simulink model "gain_scheduling_sm_2_lookuptable_WP5_seno_frequenza_1"  (R2023b)
settings: Solver=VariableStepAuto  StartTime=0.0  StopTime=10  RelTol=1e-3
values from neighbouring files (symbols this model uses):
  k1_sigma = [k1_sigma,double(subs(gains.k1, 'sigma', i))]    [gain_sheduling_WP5.m]
  k2_sigma = [k2_sigma,double(subs(gains.k2, 'sigma', i))]    [gain_sheduling_WP5.m]
  sigma = input(1)    [GS_compute_gains_LQI.m]    (also in GS_compute_gains_LQR.m; GS_compute_gains_PP.m = rif; compute_gains_WP5.m = rif; gain_sheduling_WP5.m = [-pi+pi/16:pi/16:pi])
settings Model: Creator=miche  LastModifiedBy=miche

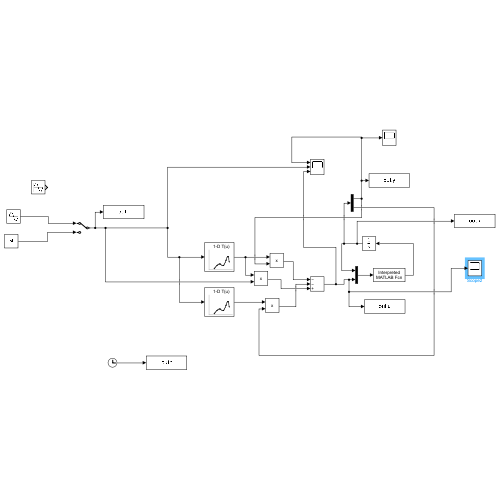
[thumbnail: Simulink's stored preview of the top-level diagram]
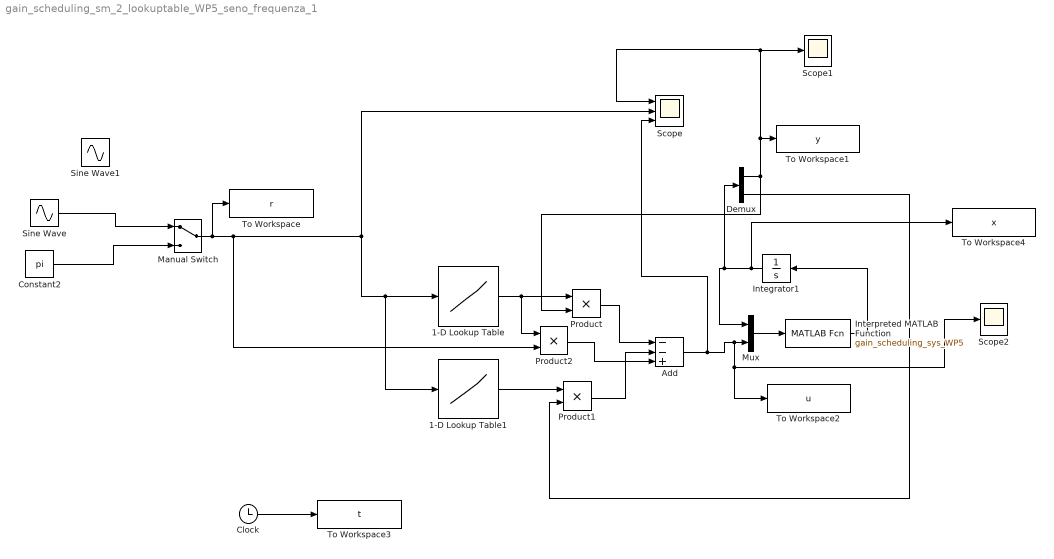
== system gain_scheduling_sm_2_lookuptable_WP5_seno_frequenza_1 ==
  1-D Lookup Table : Lookup_n-D  NumberOfTableDimensions=1  BreakpointsForDimension1=sigma  Table=k1_sigma  InterpMethod=Cubic spline  InternalRulePriority=Speed  RndMeth=Simplest
  1-D Lookup Table1 : Lookup_n-D  NumberOfTableDimensions=1  BreakpointsForDimension1=sigma  Table=k2_sigma  InterpMethod=Cubic spline  InternalRulePriority=Speed  RndMeth=Simplest
  Add : Sum  Inputs=--+
  Clock : Clock
  Constant2 : Constant  Value=pi
  Demux : Demux  Outputs=2
  Integrator1 : Integrator
  Interpreted MATLAB Function : MATLABFcn  MATLABFcn=gain_scheduling_sys_WP5  OutputDimensions=2
  Manual Switch : ManualSwitch
  Mux : Mux  Inputs=2
  Product : Product
  Product1 : Product
  Product2 : Product
  Scope : Scope  NumInputPorts=3
  Scope1 : Scope
  Scope2 : Scope
  Sine Wave : Sin  Amplitude=3.14  SampleTime=0
  Sine Wave1 : Sin  SampleTime=0
  To Workspace : ToWorkspace  VariableName=r  SampleTime=-1
  To Workspace1 : ToWorkspace  VariableName=y  SampleTime=-1
  To Workspace2 : ToWorkspace  VariableName=u  SampleTime=-1
  To Workspace3 : ToWorkspace  VariableName=t  SampleTime=-1
  To Workspace4 : ToWorkspace  VariableName=x  SampleTime=-1
  wires:
  Interpreted MATLAB Function/1 -> Integrator1/1
  1-D Lookup Table/1 -> Product2/1, Product/1
  1-D Lookup Table1/1 -> Product1/1
  Manual Switch/1 -> To Workspace/1, Product2/2, 1-D Lookup Table1/1, 1-D Lookup Table/1, Scope/2
  Integrator1/1 -> To Workspace4/1, Demux/1, Mux/1
  Add/1 -> Scope/3, To Workspace2/1, Scope2/1, Mux/2
  Mux/1 -> Interpreted MATLAB Function/1
  Constant2/1 -> Manual Switch/2
  Demux/1 -> Scope/1, Scope1/1, To Workspace1/1, Product/2
  Demux/2 -> Product1/2
  Product2/1 -> Add/3
  Product/1 -> Add/1
  Product1/1 -> Add/2
  Sine Wave/1 -> Manual Switch/1
  Clock/1 -> To Workspace3/1
